simulink model "theta_model_validation"  (R2025a)
settings: Solver=FixedStepAuto  StartTime=0.0  StopTime=30  FixedStep=0.002  RelTol=1e-3
PreLoadFcn:
  | d=fileparts(get_param('theta_model_validation','FileName')); while ~isempty(d)&&~isfile(fullfile(d,'setup_paths.m')), n=fileparts(d); if strcmp(n,d),break;end; d=n; end; if isfile(fullfile(d,'setup_paths.m')), addpath(d); setup_paths; end
  | Ensamblaje_pendulo_furuta_multibody_v4_DataFile;
InitFcn:
  | Ensamblaje_pendulo_furuta_multibody_v4_DataFile;
model workspace: external: MATLAB File C:\Users\sebas\Documents\TESIS\Scape\Ensamblaje_pendulo_furuta_multibody_v4_DataFile.m (data not in the file)
libraries: fl_lib x6, nesl_utility x6, sm_lib x2, ee_lib x1, quarc_library x1
settings Model: Creator=sebas  LastModifiedBy=sebas
settings ExplorerConfigSet: InternalSimMechanicsExplorerSettings=|
  | <ExplorerConfiguration>
  | 
  |   <canonicalview>planar_xy</canonicalview>
  | 
  |   <TilePanel>
  |     <TileInfo>
  |       <Tiles Columns="1" Count="1" Height="592" Rows="1" Width="1064">
  |         <Row Weight="1"/>
  |         <Column Weight="1"/>
  |         <Tile Height="1" Width="1" X="0" Y="0"/>
  |       </Tiles>
  |     </TileInfo>
  |     <SceneInfo>
  |       <SceneViewer>
  |         <IsThisViewStd>
  |           <IsStandardView>off</IsStandardView>
  |           <StandardViewName>Front</StandardViewName>
  |         </IsThisViewStd>
  |         <BGColor>
  |           <R>1</R>
  |           <G>1</G>
  |           <B>1</B>
  |           <A>1</A>
  |         </BGColor>
  |         <Camera>
  |           <DoPerspective>off</DoPerspective>
  |           <Position>
  |             <X>0.15562955258539984</X>
  |             <Y>0.44865320150635074</Y>
  |             <Z>-0.59717677203901176</Z>
  |           </Position>
  |           <Center>
  |             <X>-0.047110070178558651</X>
  |             <Y>0.055245833996093285</Y>
  |             <Z>0.019492845057677309</Z>
  |           </Center>
  |           <Up>
  |             <X>-0.56022370531309607</X>
  |             <Y>0.7694686491141598</Y>
  |             <Z>0.30670408871695148</Z>
  |           </Up>
  |           <XLim>0.11928668495035986</XLim>
  |           <YLim>0.11928668495035986</YLim>
  |           <ViewLimDist>0.01</ViewLimDist>
  |         </Camera>
  |       </SceneViewer>
  |     </SceneInfo>
  |   </TilePanel>
  | 
  |   <MechEditorPanel>
  |     <GfxPanelCameraMap/>
  |     <Cameras/>
  |     <VideoCreator>
  |       <IncludeTiles>All</IncludeTiles>
  |       <IncludeTime>on</IncludeTime>
  |       <IncludeWorldFrame>off</IncludeWorldFrame>
  |       <PlaybackSpeedRatio>1</PlaybackSpeedRatio>
  |       <FrameRate>30</FrameRate>
  |       <FrameSize>auto</FrameSize>
  |       <VideoFormat>UncompressedAVI</VideoFormat>
  |     </VideoCreator>
  |   </MechEditorPanel>
  | 
  |   <PlaybackSettings>
  |     <PlaybackSpeedFactor>1</PlaybackSpeedFactor>
  |   </PlaybackSettings>
  | 
  | </ExplorerConfiguration>

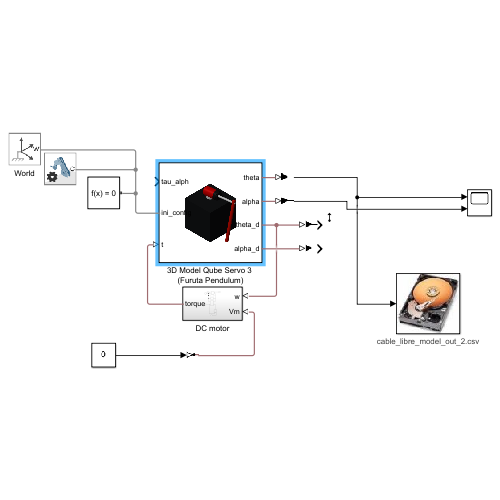
[thumbnail: Simulink's stored preview of the top-level diagram]
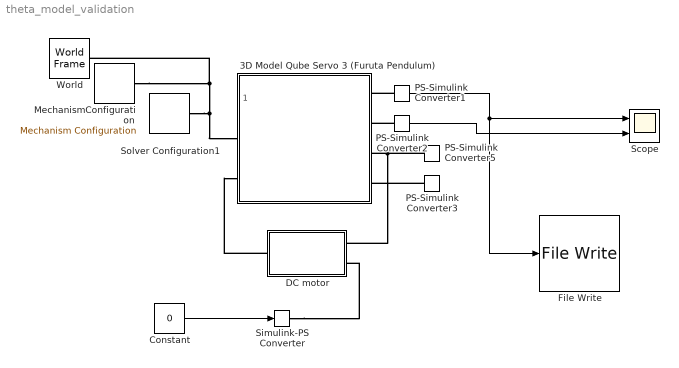
== system theta_model_validation ==
  3D Model Qube Servo 3 (Furuta Pendulum) : Subsystem  ReferencedSubsystem=Model3d_Furuta_Pendulum
      settings: PortSchema="{\"entries\":[{\"content\":{\"sides\":[{\"content\":{\"connectorIds\":[\"In1\",\"LConn1\",\"RConn1\"]},\"type\":\"ConnectorPlacement.EquallySpacedRectSide\",\"uuid\":\"a4687828-c9dc-4620-89f9-70fc520029b1\"},{\"content\":{\"connectorIds\":[\"RConn2\",\"RConn3\",\"RConn4\",\"RConn5\"],\"side\":\"RIGHT\"},\"type\":\"ConnectorPlacement.EquallySpacedRectSide\",\"uuid\":\"21a6a3f8-f9ca-4875-ad02-4f645e066fb2\"},{\"content\":{\"side\":\"TOP\"},\"type\":\"ConnectorPlacement.EquallySpacedRectSide\",\"uuid\":\"b064abef-f9ef-4dd8-a3db-595c6ba7d55c\"}]},\"type\":\"ConnectorPlacement.EquallySpacedConnector\",\"uuid\":\"310dfd22-cc79-4c6a-8ca3-9ebbca52c939\"}],\"packageUris\":[\"http://schema.mathworks.com/mf0/Connector/R2020b\"],\"version\":\"1.0\"}"
  Constant : Constant  Value=0
  DC motor : Subsystem
  File Write : quarc_library/Sinks/To Target/File Write  source=Specify via dialog (do not evaluate)  file_name=cable_libre_model_out_2.csv  variable_name=theta  decimation=1  sample_time=-1  file_format=CSV-file  options=No header or footer  append=off  encoding=Default  bitrate=0
      settings: AttributesFormatString=%<file_name>  SourceProductName=QUARC Targets
  MechanismConfiguration : sm_lib/Utilities/Mechanism Configuration  UniformGravity=Constant  GravityVector=[0 -9.7807 0]  GravityVectorUnits=m/s^2  LinearizationDelta=0.001  JointModeTransitionNonlinearIterations=2
  PS-Simulink Converter{1..3,5} (4 alike) : nesl_utility/PS-Simulink Converter  PhysicalDomain=network_engine_domain  SubClassName=ps_output  LeftPortType=input  RightPortType=output  PseudoPeriodic=off  Frequencies=[]  VectorFormat=inherit  Unit=inherit  AffineConversion=off
  Scope : Scope  NumInputPorts=2
      settings: ActiveDisplayYMinimum=-1.8228145221609748  ActiveDisplayYMaximum=0.69736743149980884  DataLoggingVariableName=ScopeData8
  Simulink-PS Converter : nesl_utility/Simulink-PS Converter  PhysicalDomain=network_engine_domain  SubClassName=ps_input  LeftPortType=input  RightPortType=output  PseudoPeriodic=off  Frequencies=[]  NoiseDistribution=none  NoiseParameters=[]  Unit=1  AffineConversion=off  FilteringAndDerivatives=filter  SimscapeFilterOrder=1  InputFilterTimeConstant=0.001  UdotUserProvided=0
  Solver Configuration1 : nesl_utility/Solver Configuration  PhysicalDomain=network_engine_domain  SubClassName=solver  LeftPortType=input  RightPortType=generic  Tones=[]  Harmonics=[]  SimulateNoise=off  Profile=off  UseLocalSampling=off  EnableSwitchedLinearOptims=on  FrequencyDomain=off  UseCCode=off  RelTol=0.001  AbsTol=0.001  MinStep=1e-09  ToWorkspace=off  RevertToSquareIcSolve=off  NumHomotopyIterations=100  PhasorMode=off  PhasorModeNumHarmonics=1  ConsistencySolver=NEWTON_XTOL_AFTER_FTOL  IndexReductionMethod=DerivativeReplacement  DoDC=off  ResidualTolerance=1e-09  ConsistencyTolSource=GLOBAL  ConsistencyAbsTol=0.001  ConsistencyRelTol=0.001  ConsistencyTolFactor=1e-9  UseLocalSolver=off  LocalSolverChoice=NE_BACKWARD_EULER_ADVANCER  ResolveIndetEquations=on  FunctionEvalNumThread=1  LocalSolverSampleTime=0.002  DoFixedCost=on  MaxNonlinIter=5  MaxModeIter=2  ComputeImpulses=on  ImpulseIterations=2  LinearAlgebra=auto  LinearAlgebraNumThread=0  EquationFormulation=NE_TIME_EF  DelaysMemoryBudget=1024  AutomaticFiltering=on  FilteringTimeConstant=0.001  PartitionStorageMethod=AS_NEEDED  PartitionMemoryBudget=1024  PartitionMethod=ROBUST  MultibodyUseLocalSolver=off  MultibodyLocalSolverChoice=ODE1  MultibodyLocalSolverSampleTime=0.002
  World : sm_lib/Frames and Transforms/World Frame
  wires:
  PS-Simulink Converter2/1 -> Scope/2
  PS-Simulink Converter1/1 -> File Write/1, Scope/1
  Constant/1 -> Simulink-PS Converter/1
  connections:
  MechanismConfiguration/RConn1 -- Solver Configuration1/RConn1 -- 3D Model Qube Servo 3 (Furuta Pendulum)/LConn1 -- World/RConn1
  PS-Simulink Converter1/LConn1 -- 3D Model Qube Servo 3 (Furuta Pendulum)/RConn2
  PS-Simulink Converter2/LConn1 -- 3D Model Qube Servo 3 (Furuta Pendulum)/RConn3
  DC motor/LConn1 -- 3D Model Qube Servo 3 (Furuta Pendulum)/RConn1
  Simulink-PS Converter/RConn1 -- DC motor/RConn2
  PS-Simulink Converter3/LConn1 -- 3D Model Qube Servo 3 (Furuta Pendulum)/RConn5
  PS-Simulink Converter5/LConn1 -- DC motor/RConn1 -- 3D Model Qube Servo 3 (Furuta Pendulum)/RConn4

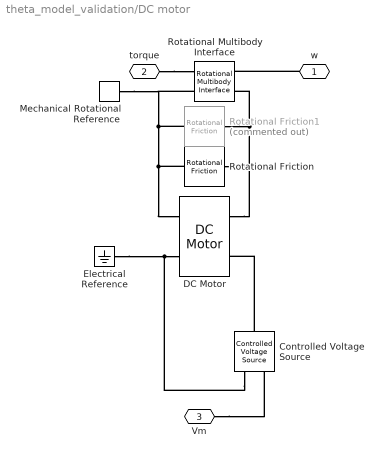
== system theta_model_validation/DC motor ==
  Controlled Voltage Source : fl_lib/Electrical/Electrical Sources/Controlled Voltage Source
  DC Motor : ee_lib/Electromechanical/Brushed Motors/DC Motor  field_option=ee.enum.field_option.pm  Rf=100 Ohm  Lf=1 H  Laf=0.15 H  If0=0 A  parameterization=ee.enum.dcparam_option.circuit_param  Ra=7.5 Ohm  La=1.15e-3 H  emf_or_torque=ee.enum.emf_or_torque.kv  Kv=0.0422 V*s/rad  Ki=0.0422 N*m/A  T_stall=0.24e-3 N*m  w_max=5400 rpm  w_rated=4579 rpm  P_rated=9.8 W  V_rated=24 V  lam_param=ee.enum.lam_param.damping  i_noload=16 mA  V_i_noload=24 V  J=1.4e-6 kg*m^2  lam=4.8390e-6 N*m*s/rad  speed0=0 rpm  alpha=3.93e-3 1/K  Tmeas=25 degC  thermal_mass=100 J/K  initial_temperature=25 degC
  Electrical Reference : fl_lib/Electrical/Electrical Elements/Electrical Reference
  Mechanical Rotational Reference : fl_lib/Mechanical/Rotational Elements/Mechanical Rotational Reference
  Rotational Friction : fl_lib/Mechanical/Rotational Elements/Rotational Friction  brkwy_trq=0*2.910555e-05+1*4.081637e-05 N*m  brkwy_vel=1.082312e-02 rad/s  Col_trq=2.910555e-05 N*m  visc_coef=0 N*m*s/rad  w_specify=off  w_priority=None  w=0 rad/s  w_nominal_specify=off  w_nominal_value=1  w_nominal_unit=rad/s  t_specify=off  t_priority=None  t=0 N*m  t_nominal_specify=off  t_nominal_value=1  t_nominal_unit=N*m
  Rotational Friction1 : fl_lib/Mechanical/Rotational Elements/Rotational Friction  Commented=on  brkwy_trq=7.066e-04 N*m  brkwy_vel=0.1 rad/s  Col_trq=7.066e-09 N*m  visc_coef=0 N*m*s/rad  w_specify=off  w_priority=None  w=0 rad/s  w_nominal_specify=off  w_nominal_value=1  w_nominal_unit=rad/s  t_specify=off  t_priority=None  t=0 N*m  t_nominal_specify=off  t_nominal_value=1  t_nominal_unit=N*m
  Rotational Multibody Interface : fl_lib/Mechanical/Multibody Interfaces/Rotational Multibody Interface
  w : PMIOPort  Side=Right
  torque : PMIOPort  Port=2  Side=Left
  Vm : PMIOPort  Port=3  Side=Right
  connections:
  Rotational Friction/LConn1 -- DC Motor/LConn2 -- Rotational Friction1/LConn1 -- Rotational Multibody Interface/RConn2
  torque/RConn1 -- Rotational Multibody Interface/LConn1
  Rotational Friction/RConn1 -- Rotational Friction1/RConn1 -- Rotational Multibody Interface/LConn2 -- Mechanical Rotational Reference/LConn1 -- DC Motor/RConn2
  Vm/RConn1 -- Controlled Voltage Source/RConn1
  w/RConn1 -- Rotational Multibody Interface/RConn1
  DC Motor/RConn1 -- Electrical Reference/LConn1 -- Controlled Voltage Source/RConn2
  Controlled Voltage Source/LConn1 -- DC Motor/LConn1
